simulink model "n7_feedback_linearization_VSC_controller"  (R2023b)
settings: Solver=VariableStepAuto  StartTime=0.0  StopTime=20  RelTol=1e-3
values from neighbouring files (symbols this model uses):
  alfa_prime = beta_prime*A_tilde    [n0_collaborative_class_main.m]    (also in svc_robot.m = beta_prime*A)
  alfa_prime_contr = beta_prime_contr*F_contr    [n0_collaborative_class_main.m]
  beta_prime = [p^3 3*p^2 3*p 1]    [n0_collaborative_class_main.m]    (also in svc_robot.m)
  beta_prime_contr = flip(poly([p_contr p_contr p_contr p_contr]))    [n0_collaborative_class_main.m]
  BI = 0.02    [n0_collaborative_class_main.m]    (also in svc_robot.m)
  dx_0 = [0;1;0;1]*0.01    [n0_collaborative_class_main.m]    (also in svc_robot.m = [0;1;0;1]*0.1)
  gamma = beta3/b4    [n0_collaborative_class_main.m]    (also in svc_robot.m)
  gamma_contr = beta3_contr/b4_contr    [n0_collaborative_class_main.m]
  M = 1    [n0_collaborative_class_main.m]    (also in svc_robot.m)
  q = 1    [collaborative_class_main.m]    (also in n0_collaborative_class_main.m = 20; svc_robot.m = 20)
  r = 100    [collaborative_class_main.m]    (also in n0_collaborative_class_main.m = 0.7; svc_robot.m = 0.7)
  T = Mr_contr*Mr^-1    [n0_collaborative_class_main.m]    (also in svc_robot.m = Mr_tilde*Mr^-1)
  u_bar = m*g*l*cos(x2_bar)    [collaborative_class_main.m]    (also in n0_collaborative_class_main.m; svc_robot.m)
  W = 2    [n0_collaborative_class_main.m]    (also in svc_robot.m)
  x2_bar = pi/4    (= 0.785398163397)    [collaborative_class_main.m]    (also in n0_collaborative_class_main.m; svc_robot.m)
settings Model: Creator=Kevin  LastModifiedBy=teoma

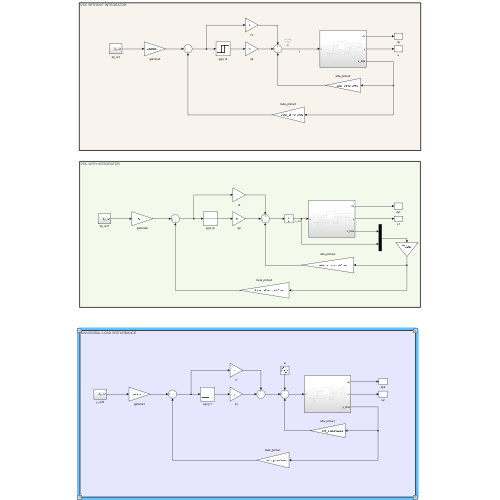
[thumbnail: Simulink's stored preview of the top-level diagram]
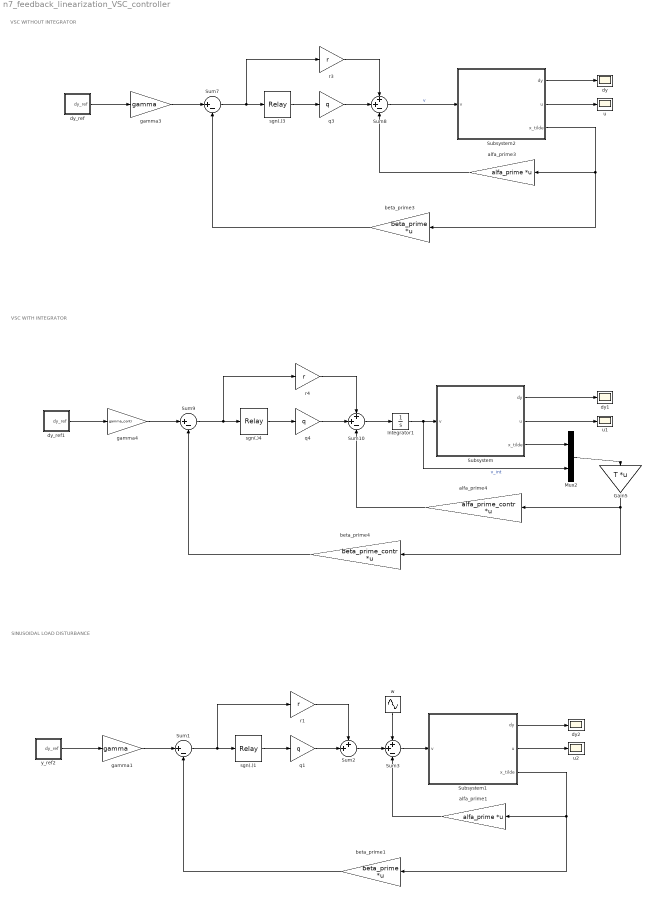
== system n7_feedback_linearization_VSC_controller ==
  note: VSC WITH INTEGRATOR
  note: VSC WITHOUT INTEGRATOR
  note: SINUSOIDAL LOAD DISTURBANCE
  Gain5 : Gain  Gain=T  Multiplication=Matrix(K*u) (u vector)
  Integrator1 : Integrator
  Mux2 : Mux  Inputs=2
  Subsystem : Subsystem
  Subsystem1 : Subsystem
  Subsystem2 : Subsystem
  Sum1 : Sum  Inputs=|+-
  Sum10 : Sum  Inputs=++-
  Sum2 : Sum  Inputs=++|
  Sum3 : Sum  Inputs=++-
  Sum7 : Sum  Inputs=|+-
  Sum8 : Sum  Inputs=++-
  Sum9 : Sum  Inputs=|+-
  alfa_prime1 : Gain  Gain=alfa_prime  Multiplication=Matrix(K*u) (u vector)
  alfa_prime3 : Gain  Gain=alfa_prime  Multiplication=Matrix(K*u) (u vector)
  alfa_prime4 : Gain  Gain=alfa_prime_contr  Multiplication=Matrix(K*u) (u vector)
  beta_prime1 : Gain  Gain=beta_prime  Multiplication=Matrix(K*u) (u vector)
  beta_prime3 : Gain  Gain=beta_prime  Multiplication=Matrix(K*u) (u vector)
  beta_prime4 : Gain  Gain=beta_prime_contr  Multiplication=Matrix(K*u) (u vector)
  dy : Scope
  dy1 : Scope
  dy2 : Scope
  dy_ref : Subsystem
  dy_ref1 : Subsystem
  gamma1 : Gain  Gain=gamma
  gamma3 : Gain  Gain=gamma
  gamma4 : Gain  Gain=gamma_contr
  q1 : Gain  Gain=q
  q3 : Gain  Gain=q
  q4 : Gain  Gain=q
  r1 : Gain  Gain=r
  r3 : Gain  Gain=r
  r4 : Gain  Gain=r
  sgn(.)1 : Relay  OnSwitchValue=BI/2  OffSwitchValue=-BI/2  OnOutputValue=M  OffOutputValue=-M
  sgn(.)3 : Relay  OnSwitchValue=BI/2  OffSwitchValue=-BI/2  OnOutputValue=M  OffOutputValue=-M
  sgn(.)4 : Relay  OnSwitchValue=BI/2  OffSwitchValue=-BI/2  OnOutputValue=M  OffOutputValue=-M
  u : Scope
  u1 : Scope
  u2 : Scope
  w : Sin  Amplitude=W  Frequency=5  SampleTime=0
  y_ref2 : Subsystem
  wires:
  alfa_prime3/1 -> Sum8/3
  r3/1 -> Sum8/1
  beta_prime3/1 -> Sum7/2
  Sum7/1 -> r3/1, sgn(.)3/1
  gamma3/1 -> Sum7/1
  q3/1 -> Sum8/2
  Sum8/1 -> Subsystem2/1(v)  "v"
  sgn(.)3/1 -> q3/1
  Subsystem2/3(x_tilde) -> beta_prime3/1, alfa_prime3/1
  Subsystem2/2(u) -> u/1
  alfa_prime4/1 -> Sum10/3
  q4/1 -> Sum10/2
  Mux2/1 -> Gain5/1
  gamma4/1 -> Sum9/1
  sgn(.)4/1 -> q4/1
  r4/1 -> Sum10/1
  Sum10/1 -> Integrator1/1
  Integrator1/1 -> Subsystem/1(v), Mux2/2  "v_int"
  Sum9/1 -> r4/1, sgn(.)4/1
  beta_prime4/1 -> Sum9/2
  Subsystem/3(x_tilde) -> Mux2/1
  Subsystem/1(dy) -> dy1/1
  Gain5/1 -> beta_prime4/1, alfa_prime4/1
  Subsystem/2(u) -> u1/1
  Subsystem2/1(dy) -> dy/1
  dy_ref/1(dy_ref) -> gamma3/1
  dy_ref1/1(dy_ref) -> gamma4/1
  Subsystem1/3(x_tilde) -> beta_prime1/1, alfa_prime1/1
  q1/1 -> Sum2/2
  beta_prime1/1 -> Sum1/2
  sgn(.)1/1 -> q1/1
  r1/1 -> Sum2/1
  Subsystem1/1(dy) -> dy2/1
  gamma1/1 -> Sum1/1
  Sum1/1 -> r1/1, sgn(.)1/1
  Subsystem1/2(u) -> u2/1
  y_ref2/1(dy_ref) -> gamma1/1
  Sum3/1 -> Subsystem1/1(v)
  w/1 -> Sum3/1
  Sum2/1 -> Sum3/2
  alfa_prime1/1 -> Sum3/3

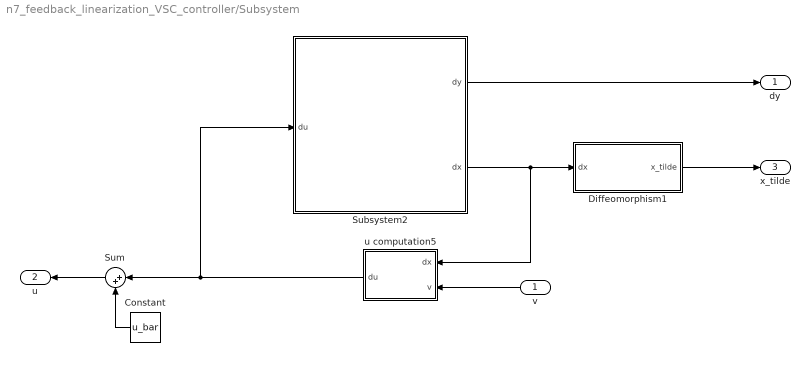
== system n7_feedback_linearization_VSC_controller/Subsystem ==
  v : Inport
  Constant : Constant  Value=u_bar
  Diffeomorphism1 : MATLAB Function  TreatAsAtomicUnit=on
  Subsystem2 : Subsystem
  Sum : Sum  Inputs=|++
  u computation5 : MATLAB Function  TreatAsAtomicUnit=on
  dy : Outport
  u : Outport  Port=2
  x_tilde : Outport  Port=3
  wires:
  v/1 -> u computation5/2(v)
  Diffeomorphism1/1(x_tilde) -> x_tilde/1
  Subsystem2/2(dx) -> Diffeomorphism1/1(dx), u computation5/1(dx)
  u computation5/1(du) -> Sum/1, Subsystem2/1(du)
  Sum/1 -> u/1
  Constant/1 -> Sum/2
  Subsystem2/1(dy) -> dy/1

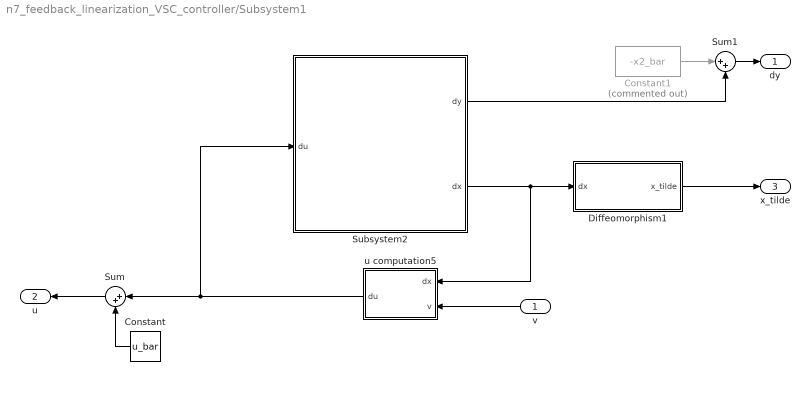
== system n7_feedback_linearization_VSC_controller/Subsystem1 ==
  v : Inport
  Constant : Constant  Value=u_bar
  Constant1 : Constant  Commented=on  Value=-x2_bar
  Diffeomorphism1 : MATLAB Function  TreatAsAtomicUnit=on
  Subsystem2 : Subsystem
  Sum : Sum  Inputs=|++
  Sum1 : Sum  Inputs=|++
  u computation5 : MATLAB Function  TreatAsAtomicUnit=on
  dy : Outport
  u : Outport  Port=2
  x_tilde : Outport  Port=3
  wires:
  v/1 -> u computation5/2(v)
  Diffeomorphism1/1(x_tilde) -> x_tilde/1
  Subsystem2/2(dx) -> Diffeomorphism1/1(dx), u computation5/1(dx)
  Subsystem2/1(dy) -> Sum1/2
  u computation5/1(du) -> Sum/1, Subsystem2/1(du)
  Sum/1 -> u/1
  Constant/1 -> Sum/2
  Constant1/1 -> Sum1/1
  Sum1/1 -> dy/1

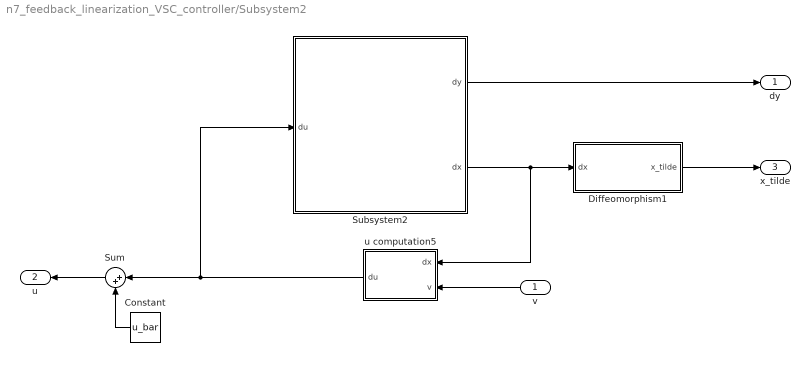
== system n7_feedback_linearization_VSC_controller/Subsystem2 ==
  v : Inport
  Constant : Constant  Value=u_bar
  Diffeomorphism1 : MATLAB Function  TreatAsAtomicUnit=on
  Subsystem2 : Subsystem
  Sum : Sum  Inputs=|++
  u computation5 : MATLAB Function  TreatAsAtomicUnit=on
  dy : Outport
  u : Outport  Port=2
  x_tilde : Outport  Port=3
  wires:
  v/1 -> u computation5/2(v)
  Diffeomorphism1/1(x_tilde) -> x_tilde/1
  Subsystem2/2(dx) -> Diffeomorphism1/1(dx), u computation5/1(dx)
  Subsystem2/1(dy) -> dy/1
  u computation5/1(du) -> Sum/1, Subsystem2/1(du)
  Sum/1 -> u/1
  Constant/1 -> Sum/2

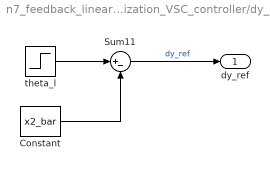
== system n7_feedback_linearization_VSC_controller/dy_ref ==
  Constant : Constant  Value=x2_bar
  Sum11 : Sum  Inputs=|+-
  theta_l : Step  After=pi/4  SampleTime=0
  dy_ref : Outport
  wires:
  theta_l/1 -> Sum11/1
  Sum11/1 -> dy_ref/1  "dy_ref"
  Constant/1 -> Sum11/2

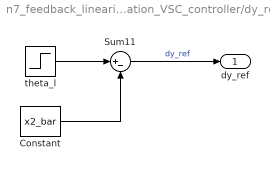
== system n7_feedback_linearization_VSC_controller/dy_ref1 ==
  Constant : Constant  Value=x2_bar
  Sum11 : Sum  Inputs=|+-
  theta_l : Step  After=pi/4  SampleTime=0
  dy_ref : Outport
  wires:
  theta_l/1 -> Sum11/1
  Sum11/1 -> dy_ref/1  "dy_ref"
  Constant/1 -> Sum11/2

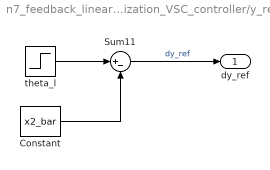
== system n7_feedback_linearization_VSC_controller/y_ref2 ==
  Constant : Constant  Value=x2_bar
  Sum11 : Sum  Inputs=|+-
  theta_l : Step  After=pi/4  SampleTime=0
  dy_ref : Outport
  wires:
  theta_l/1 -> Sum11/1
  Sum11/1 -> dy_ref/1  "dy_ref"
  Constant/1 -> Sum11/2

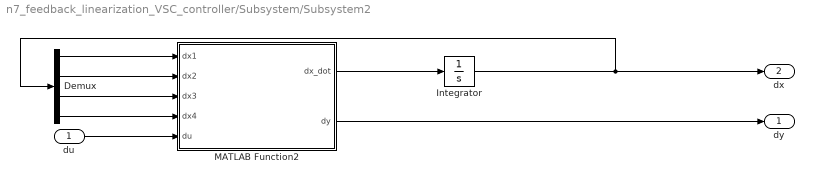
== system n7_feedback_linearization_VSC_controller/Subsystem/Subsystem2 ==
  du : Inport
  Demux : Demux
  Integrator : Integrator  InitialCondition=dx_0
  MATLAB Function2 : MATLAB Function  TreatAsAtomicUnit=on
  dy : Outport
  dx : Outport  Port=2
  wires:
  Integrator/1 -> Demux/1, dx/1
  du/1 -> MATLAB Function2/5(du)
  MATLAB Function2/2(dy) -> dy/1
  MATLAB Function2/1(dx_dot) -> Integrator/1
  Demux/1 -> MATLAB Function2/1(dx1)
  Demux/2 -> MATLAB Function2/2(dx2)
  Demux/3 -> MATLAB Function2/3(dx3)
  Demux/4 -> MATLAB Function2/4(dx4)

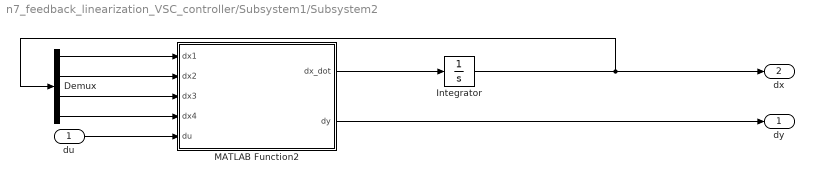
== system n7_feedback_linearization_VSC_controller/Subsystem1/Subsystem2 ==
  du : Inport
  Demux : Demux
  Integrator : Integrator  InitialCondition=dx_0
  MATLAB Function2 : MATLAB Function  TreatAsAtomicUnit=on
  dy : Outport
  dx : Outport  Port=2
  wires:
  Integrator/1 -> Demux/1, dx/1
  du/1 -> MATLAB Function2/5(du)
  MATLAB Function2/2(dy) -> dy/1
  MATLAB Function2/1(dx_dot) -> Integrator/1
  Demux/1 -> MATLAB Function2/1(dx1)
  Demux/2 -> MATLAB Function2/2(dx2)
  Demux/3 -> MATLAB Function2/3(dx3)
  Demux/4 -> MATLAB Function2/4(dx4)

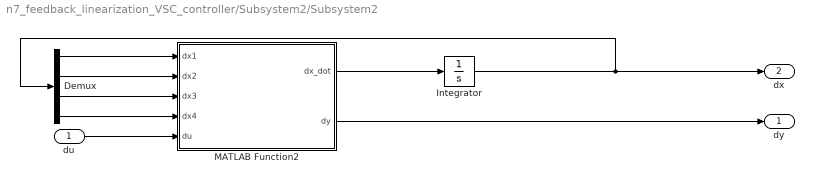
== system n7_feedback_linearization_VSC_controller/Subsystem2/Subsystem2 ==
  du : Inport
  Demux : Demux
  Integrator : Integrator  InitialCondition=dx_0
  MATLAB Function2 : MATLAB Function  TreatAsAtomicUnit=on
  dy : Outport
  dx : Outport  Port=2
  wires:
  Integrator/1 -> Demux/1, dx/1
  du/1 -> MATLAB Function2/5(du)
  MATLAB Function2/2(dy) -> dy/1
  MATLAB Function2/1(dx_dot) -> Integrator/1
  Demux/1 -> MATLAB Function2/1(dx1)
  Demux/2 -> MATLAB Function2/2(dx2)
  Demux/3 -> MATLAB Function2/3(dx3)
  Demux/4 -> MATLAB Function2/4(dx4)

== matlab function n7_feedback_linearization_VSC_controller/Subsystem2/Diffeomorphism1 ==
  data: dx input; x_tilde output
function x_tilde  = fcn(dx)

dx1 = dx(1);
dx2 = dx(2);
dx3 = dx(3);
dx4 = dx(4);
k = 0.8;
Jm = 4e-4;
Jl= 4e-4;
Bm = 0.015;
Bl = 0;
m = 0.3;
l = 0.3;
g = 9.81;

x1_tilde = -dx2;
x2_tilde = -dx1;
x3_tilde = (k*(pi/4 + dx2))/Jl - (k*(dx4 + sqrt(2)/2*m*g*l/k+pi/4))/Jl + (g*l*m*cos(pi/4 + dx2))/Jl;
x4_tilde = (k*dx1)/Jl - (k*dx3)/Jl - (g*l*m*sin(pi/4 + dx2)*dx1)/Jl;

x_tilde = zeros(length(dx),1);
x_tilde(1) = x1_tilde;
x_tilde(2) = x2_tilde;
x_tilde(3) = x3_tilde;
x_tilde(4) = x4_tilde;

== matlab function n7_feedback_linearization_VSC_controller/Subsystem2/Subsystem2/MATLAB Function2 ==
  data: dx1 input; dx2 input; dx3 input; dx4 input; du input; dx_dot output; dy output
function [dx_dot, dy]  = fcn(dx1,dx2,dx3,dx4, du)

k = 0.8;
Jm = 4e-4;
Jl= 4e-4;
Bm = 0.015;
Bl = 0;
m = 0.3;
l = 0.3;
g = 9.81;
x1_bar = 0;
x2_bar = pi/4;
x3_bar = 0;
x4_bar = m*g*l*cos(x2_bar)/k + x2_bar;
u_bar= m*g*l*cos(x2_bar);


dx1_dot = -k/Jl*(dx2+x2_bar)-m*g*l/Jl*(cos(dx2+x2_bar))+k/Jl*(dx4+x4_bar);
dx2_dot = dx1+x1_bar;
dx3_dot = k/Jm*(dx2+x2_bar)-Bm/Jm*(dx3+x3_bar)-k/Jm*(dx4+x4_bar)+1/Jm*(du+u_bar);
dx4_dot = dx3+x3_bar;
dy = pi/4 - (dx2+x2_bar);

dx_dot = zeros(1,4);
dx_dot(1) = dx1_dot;
dx_dot(2) = dx2_dot;
dx_dot(3) = dx3_dot;
dx_dot(4) = dx4_dot;

== matlab function n7_feedback_linearization_VSC_controller/Subsystem1/Diffeomorphism1 ==
  data: dx input; x_tilde output
function x_tilde  = fcn(dx)

dx1 = dx(1);
dx2 = dx(2);
dx3 = dx(3);
dx4 = dx(4);
k = 0.8;
Jm = 4e-4;
Jl= 4e-4;
Bm = 0.015;
Bl = 0;
m = 0.3;
l = 0.3;
g = 9.81;

x1_tilde = -dx2;
x2_tilde = -dx1;
x3_tilde = (k*(pi/4 + dx2))/Jl - (k*(dx4 + sqrt(2)/2*m*g*l/k+pi/4))/Jl + (g*l*m*cos(pi/4 + dx2))/Jl;
x4_tilde = (k*dx1)/Jl - (k*dx3)/Jl - (g*l*m*sin(pi/4 + dx2)*dx1)/Jl;

x_tilde = zeros(length(dx),1);
x_tilde(1) = x1_tilde;
x_tilde(2) = x2_tilde;
x_tilde(3) = x3_tilde;
x_tilde(4) = x4_tilde;

== matlab function n7_feedback_linearization_VSC_controller/Subsystem2/u computation5 ==
  data: dx input; du output; v input
function du  = fcn(dx, v)

%v = 0;
k = 0.8;
Jm = 4e-4;
Jl= 4e-4;
Bm = 0.015;
m = 0.3;
l = 0.3;
g = 9.81;

x1_bar = 0;
x2_bar = pi/4;
x3_bar = 0;
x4_bar = m*g*l*cos(x2_bar)/k + x2_bar;
u_bar= m*g*l*cos(x2_bar);

x1 = dx(1)+x1_bar;
x2 = dx(2)+x2_bar;
x3 = dx(3)+x3_bar;
x4 = dx(4)+x4_bar;

% HARDCODED
%u = Jl*Jm/k* (   -v+k^2/Jl^2*(x4-x2)     +   m*g*l*k/Jl^2*(sin(x2)*x2-cos(x2)-sin(x2)*x4)   -    m*g*l/Jl*cos(x2)*x1^2    +   m^2*g^2*l^2/(-Jl^2)*sin(x2)*cos(x2)    +   k^2/(Jl*Jm)*(x2-x4)     +   k*Bm/(Jl*Jm)*x3);

% from MATLAB INVERSION
 u = -(Jl*Jm*((g*l*m*cos(x2)*x1^2)/Jl + v - (k*((Bm*x3)/Jm - (k*x2)/Jm + (k*x4)/Jm))/Jl + (k*((k*x2)/Jl - (k*x4)/Jl + (g*l*m*cos(x2))/Jl))/Jl - (g*l*m*sin(x2)*((k*x2)/Jl - (k*x4)/Jl + (g*l*m*cos(x2))/Jl))/Jl))/k;
du = u - u_bar;

== matlab function n7_feedback_linearization_VSC_controller/Subsystem1/Subsystem2/MATLAB Function2 ==
  data: dx1 input; dx2 input; dx3 input; dx4 input; du input; dx_dot output; dy output
function [dx_dot, dy]  = fcn(dx1,dx2,dx3,dx4, du)

k = 0.8;
Jm = 4e-4;
Jl= 4e-4;
Bm = 0.015;
Bl = 0;
m = 0.3;
l = 0.3;
g = 9.81;
x1_bar = 0;
x2_bar = pi/4;
x3_bar = 0;
x4_bar = m*g*l*cos(x2_bar)/k + x2_bar;
u_bar= m*g*l*cos(x2_bar);


dx1_dot = -k/Jl*(dx2+x2_bar)-m*g*l/Jl*(cos(dx2+x2_bar))+k/Jl*(dx4+x4_bar);
dx2_dot = dx1+x1_bar;
dx3_dot = k/Jm*(dx2+x2_bar)-Bm/Jm*(dx3+x3_bar)-k/Jm*(dx4+x4_bar)+1/Jm*(du+u_bar);
dx4_dot = dx3+x3_bar;
dy = pi/4 - (dx2+x2_bar);

dx_dot = zeros(1,4);
dx_dot(1) = dx1_dot;
dx_dot(2) = dx2_dot;
dx_dot(3) = dx3_dot;
dx_dot(4) = dx4_dot;

== matlab function n7_feedback_linearization_VSC_controller/Subsystem1/u computation5 ==
  data: dx input; du output; v input
function du  = fcn(dx, v)

%v = 0;
k = 0.8;
Jm = 4e-4;
Jl= 4e-4;
Bm = 0.015;
m = 0.3;
l = 0.3;
g = 9.81;

x1_bar = 0;
x2_bar = pi/4;
x3_bar = 0;
x4_bar = m*g*l*cos(x2_bar)/k + x2_bar;
u_bar= m*g*l*cos(x2_bar);

x1 = dx(1)+x1_bar;
x2 = dx(2)+x2_bar;
x3 = dx(3)+x3_bar;
x4 = dx(4)+x4_bar;

% HARDCODED
%u = Jl*Jm/k* (   -v+k^2/Jl^2*(x4-x2)     +   m*g*l*k/Jl^2*(sin(x2)*x2-cos(x2)-sin(x2)*x4)   -    m*g*l/Jl*cos(x2)*x1^2    +   m^2*g^2*l^2/(-Jl^2)*sin(x2)*cos(x2)    +   k^2/(Jl*Jm)*(x2-x4)     +   k*Bm/(Jl*Jm)*x3);

% from MATLAB INVERSION
 u = -(Jl*Jm*((g*l*m*cos(x2)*x1^2)/Jl + v - (k*((Bm*x3)/Jm - (k*x2)/Jm + (k*x4)/Jm))/Jl + (k*((k*x2)/Jl - (k*x4)/Jl + (g*l*m*cos(x2))/Jl))/Jl - (g*l*m*sin(x2)*((k*x2)/Jl - (k*x4)/Jl + (g*l*m*cos(x2))/Jl))/Jl))/k;
du = u - u_bar;

== matlab function n7_feedback_linearization_VSC_controller/Subsystem/Diffeomorphism1 ==
  data: dx input; x_tilde output
function x_tilde  = fcn(dx)

dx1 = dx(1);
dx2 = dx(2);
dx3 = dx(3);
dx4 = dx(4);
k = 0.8;
Jm = 4e-4;
Jl= 4e-4;
Bm = 0.015;
Bl = 0;
m = 0.3;
l = 0.3;
g = 9.81;

x1_tilde = -dx2;
x2_tilde = -dx1;
x3_tilde = (k*(pi/4 + dx2))/Jl - (k*(dx4 + sqrt(2)/2*m*g*l/k+pi/4))/Jl + (g*l*m*cos(pi/4 + dx2))/Jl;
x4_tilde = (k*dx1)/Jl - (k*dx3)/Jl - (g*l*m*sin(pi/4 + dx2)*dx1)/Jl;

x_tilde = zeros(length(dx),1);
x_tilde(1) = x1_tilde;
x_tilde(2) = x2_tilde;
x_tilde(3) = x3_tilde;
x_tilde(4) = x4_tilde;

== matlab function n7_feedback_linearization_VSC_controller/Subsystem/Subsystem2/MATLAB Function2 ==
  data: dx1 input; dx2 input; dx3 input; dx4 input; du input; dx_dot output; dy output
function [dx_dot, dy]  = fcn(dx1,dx2,dx3,dx4, du)

k = 0.8;
Jm = 4e-4;
Jl= 4e-4;
Bm = 0.015;
Bl = 0;
m = 0.3;
l = 0.3;
g = 9.81;
x1_bar = 0;
x2_bar = pi/4;
x3_bar = 0;
x4_bar = m*g*l*cos(x2_bar)/k + x2_bar;
u_bar= m*g*l*cos(x2_bar);


dx1_dot = -k/Jl*(dx2+x2_bar)-m*g*l/Jl*(cos(dx2+x2_bar))+k/Jl*(dx4+x4_bar);
dx2_dot = dx1+x1_bar;
dx3_dot = k/Jm*(dx2+x2_bar)-Bm/Jm*(dx3+x3_bar)-k/Jm*(dx4+x4_bar)+1/Jm*(du+u_bar);
dx4_dot = dx3+x3_bar;
dy = pi/4 - (dx2+x2_bar);

dx_dot = zeros(1,4);
dx_dot(1) = dx1_dot;
dx_dot(2) = dx2_dot;
dx_dot(3) = dx3_dot;
dx_dot(4) = dx4_dot;

== matlab function n7_feedback_linearization_VSC_controller/Subsystem/u computation5 ==
  data: dx input; du output; v input
function du  = fcn(dx, v)

%v = 0;
k = 0.8;
Jm = 4e-4;
Jl= 4e-4;
Bm = 0.015;
m = 0.3;
l = 0.3;
g = 9.81;

x1_bar = 0;
x2_bar = pi/4;
x3_bar = 0;
x4_bar = m*g*l*cos(x2_bar)/k + x2_bar;
u_bar= m*g*l*cos(x2_bar);

x1 = dx(1)+x1_bar;
x2 = dx(2)+x2_bar;
x3 = dx(3)+x3_bar;
x4 = dx(4)+x4_bar;

% HARDCODED
%u = Jl*Jm/k* (   -v+k^2/Jl^2*(x4-x2)     +   m*g*l*k/Jl^2*(sin(x2)*x2-cos(x2)-sin(x2)*x4)   -    m*g*l/Jl*cos(x2)*x1^2    +   m^2*g^2*l^2/(-Jl^2)*sin(x2)*cos(x2)    +   k^2/(Jl*Jm)*(x2-x4)     +   k*Bm/(Jl*Jm)*x3);

% from MATLAB INVERSION
 u = -(Jl*Jm*((g*l*m*cos(x2)*x1^2)/Jl + v - (k*((Bm*x3)/Jm - (k*x2)/Jm + (k*x4)/Jm))/Jl + (k*((k*x2)/Jl - (k*x4)/Jl + (g*l*m*cos(x2))/Jl))/Jl - (g*l*m*sin(x2)*((k*x2)/Jl - (k*x4)/Jl + (g*l*m*cos(x2))/Jl))/Jl))/k;
du = u - u_bar;
